simulink model "Adaptive1"  (R2018b)
settings: Solver=FixedStepAuto  StartTime=0.0  StopTime=500  FixedStep=0.01  RelTol=1e-3  EnableMultiTasking=on
InitFcn:
  | gamma = 10;
settings Model: Creator=omid_zandi  LastModifiedBy=Arash
settings OptimizationCC: LifeSpan=inf
settings DebuggingCC: SFUnexpectedBacktrackingDiag=warning  SFNoUnconditionalDefaultTransitionDiag=warning
settings SFSimCC: SimUseLocalCustomCode=off
settings RTWCC: RTWUseLocalCustomCode=off
settings CodeAppCC: StateflowObjectComments=on
settings GRTTargetCC: TargetLangStandard=C89/C90 (ANSI)  GeneratePreprocessorConditionals=Disable all
settings ConfigComp: CovMetricSettings=dw  CovHtmlReporting=on  CovSaveCumulativeToWorkspaceVar=on  CovSaveSingleToWorkspaceVar=on  CovExternalEMLEnable=off

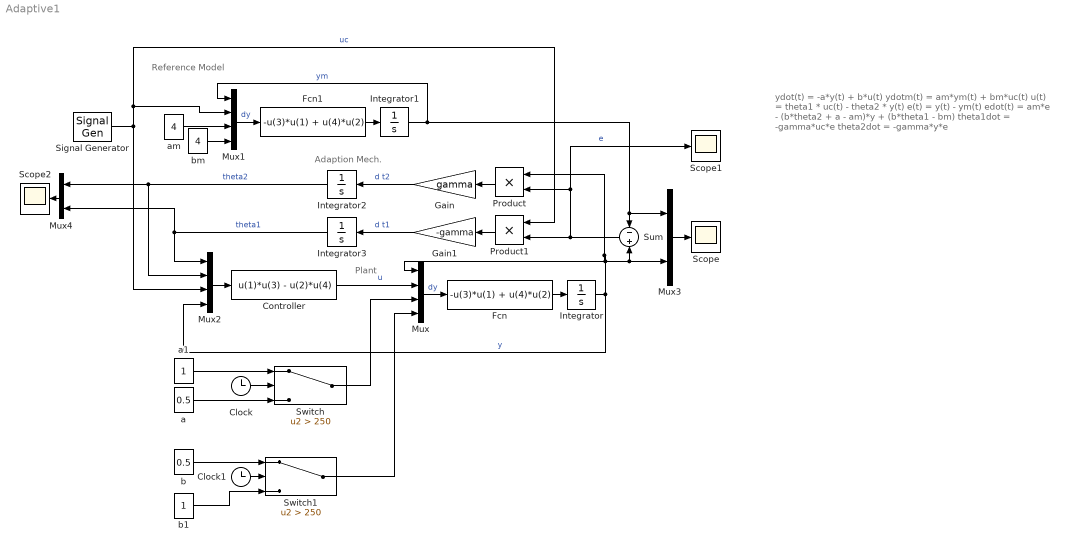
== system Adaptive1 ==
  note: ydot(t) = -a*y(t) + b*u(t)
      | ydotm(t) = am*ym(t) + bm*uc(t)
      | u(t) = theta1 * uc(t) - theta2 * y(t)
      | e(t) = y(t) - ym(t)
      | edot(t) = am*e - (b*theta2 + a - am)*y + (b*theta1 - bm)
      | theta1dot = -gamma*uc*e
      | theta2dot = -gamma*y*e
  note: Adaption Mech.
  note: Plant
  note: Reference Model
  Clock : Clock
  Clock1 : Clock
  Controller : Fcn  Expr=u(1)*u(3) - u(2)*u(4)
  Fcn : Fcn  Expr="-u(3)*u(1)  + u(4)*u(2)"
  Fcn1 : Fcn  Expr="-u(3)*u(1)  + u(4)*u(2)"
  Gain : Gain  Gain=gamma
  Gain1 : Gain  Gain=-gamma
  Integrator : Integrator  InitialCondition=randn
  Integrator1 : Integrator
  Integrator2 : Integrator
  Integrator3 : Integrator
  Mux : Mux
  Mux1 : Mux
  Mux2 : Mux
  Mux3 : Mux  Inputs=2
  Mux4 : Mux  Inputs=2
  Product : Product
  Product1 : Product
  Scope : Scope
  Scope1 : Scope
  Scope2 : Scope
  Signal Generator : SignalGenerator  WaveForm=square  Frequency=0.05
  Sum : Sum  Inputs=-|+
  Switch : Switch  Criteria=u2 > Threshold  Threshold=250
  Switch1 : Switch  Criteria=u2 > Threshold  Threshold=250
  a : Constant  Value=0.5
  a1 : Constant
  am : Constant  Value=4
  b : Constant  Value=0.5
  b1 : Constant
  bm : Constant  Value=4
  wires:
  Integrator/1 -> Product/1, Mux/1, Sum/2, Mux3/2, Mux2/4  "y"
  Controller/1 -> Mux/2  "u"
  Mux/1 -> Fcn/1  "dy"
  Fcn/1 -> Integrator/1
  Integrator1/1 -> Mux3/1, Sum/1, Mux1/1  "ym"
  Signal Generator/1 -> Product1/1, Mux1/2, Mux2/3  "uc"
  Mux1/1 -> Fcn1/1  "dy"
  Fcn1/1 -> Integrator1/1
  am/1 -> Mux1/3
  bm/1 -> Mux1/4
  Sum/1 -> Scope1/1, Product/2, Product1/2  "e"
  Mux2/1 -> Controller/1
  Integrator3/1 -> Mux2/1, Mux4/2  "theta1"
  Integrator2/1 -> Mux2/2, Mux4/1  "theta2"
  Gain/1 -> Integrator2/1  "d t2"
  Gain1/1 -> Integrator3/1  "d t1"
  Product/1 -> Gain/1
  Product1/1 -> Gain1/1
  Mux3/1 -> Scope/1
  Mux4/1 -> Scope2/1
  a/1 -> Switch/3
  a1/1 -> Switch/1
  Clock/1 -> Switch/2
  Switch/1 -> Mux/3
  Clock1/1 -> Switch1/2
  b/1 -> Switch1/1
  b1/1 -> Switch1/3
  Switch1/1 -> Mux/4
